simulink model "ros_test"  (R2025b)
settings: Solver=VariableStepAuto  StartTime=0.0  StopTime=inf  RelTol=1e-3
libraries: ros2lib x3
settings Model: Creator=vulcangrip  LastModifiedBy=cyclone

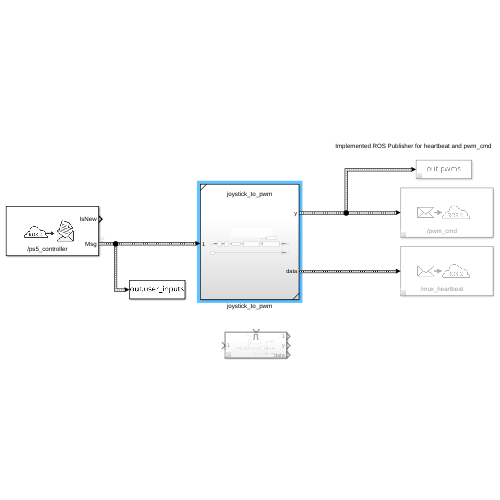
[thumbnail: Simulink's stored preview of the top-level diagram]
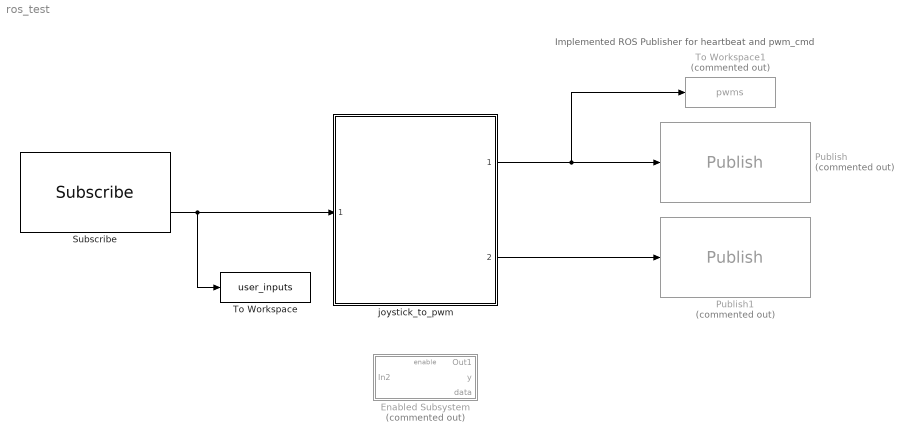
== system ros_test ==
  note: Implemented ROS Publisher for heartbeat and pwm_cmd
  Enabled Subsystem : Subsystem  Commented=on  TreatAsAtomicUnit=on
  Publish : ros2lib/Publish  Commented=on  topicSource=Specify your own  topic=/pwm_cmd  messageType=custom_interfaces/Pwms  QOSHistory=Keep last  QOSDepth=10  QOSReliability=Reliable  QOSDurability=Volatile  QOSDeadline=Inf  QOSLifespan=Inf  QOSLiveliness=Automatic  QOSLeaseDuration=Inf  QOSAvoidROSNamespaceConventions=off
  Publish1 : ros2lib/Publish  Commented=on  topicSource=Specify your own  topic=/mux_heartbeat  messageType=std_msgs/Bool  QOSHistory=Keep last  QOSDepth=10  QOSReliability=Reliable  QOSDurability=Volatile  QOSDeadline=Inf  QOSLifespan=Inf  QOSLiveliness=Automatic  QOSLeaseDuration=Inf  QOSAvoidROSNamespaceConventions=off
  Subscribe : ros2lib/Subscribe  topicSource=Specify your own  topic=/ps5_controller  messageType=remote_control_interface/Gamepad  sampleTime=1  QOSHistory=Keep last  QOSDepth=10  QOSReliability=Reliable  QOSDurability=Volatile  QOSDeadline=Inf  QOSLifespan=Inf  QOSLiveliness=Automatic  QOSLeaseDuration=Inf  QOSAvoidROSNamespaceConventions=off
  To Workspace : ToWorkspace  VariableName=user_inputs  SaveFormat=Timeseries  SampleTime=-1
  To Workspace1 : ToWorkspace  Commented=on  VariableName=pwms  SaveFormat=Timeseries  SampleTime=-1
  joystick_to_pwm : Subsystem  ReferencedSubsystem=joystick_to_pwm
  wires:
  Subscribe/2 -> To Workspace/1, joystick_to_pwm/1
  joystick_to_pwm/1 -> Publish/1, To Workspace1/1
  joystick_to_pwm/2 -> Publish1/1

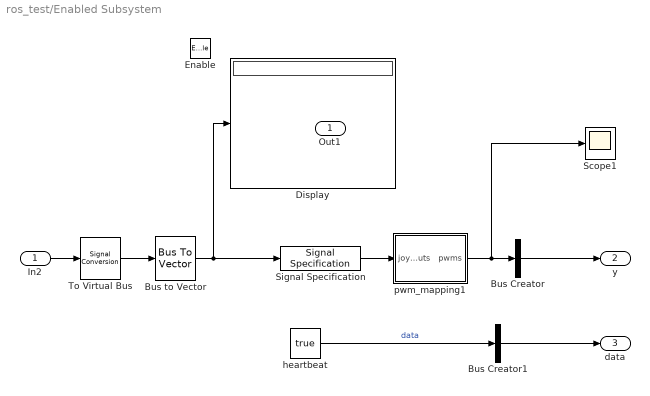
== system ros_test/Enabled Subsystem ==
  In2 : Inport
  Enable : EnablePort
  Bus Creator : BusCreator  Inputs=1  OutDataTypeStr=Bus: SL_Bus_custom_interfaces_Pwms  NonVirtualBus=on
  Bus Creator1 : BusCreator  Inputs=1  OutDataTypeStr=Bus: SL_Bus_std_msgs_Bool  NonVirtualBus=on
  Bus to Vector : BusToVector
  Display : Display
  Scope1 : Scope
      settings: ActiveDisplayYMinimum=-823919.38808281254  ActiveDisplayYMaximum=486800.61191718746
  Signal Specification : SignalSpecification  Dimensions=[6,1]
  To Virtual Bus : SignalConversion  ConversionOutput=Virtual bus  OverrideOpt=off
  heartbeat : Constant  Value=true
  pwm_mapping1 : MATLAB Function  TreatAsAtomicUnit=on
  Out1 : Outport
  y : Outport  Port=2
  data : Outport  Port=3
  wires:
  heartbeat/1 -> Bus Creator1/1  "data"
  In2/1 -> To Virtual Bus/1
  Signal Specification/1 -> pwm_mapping1/1(joystick_inputs)
  Bus to Vector/1 -> Signal Specification/1, Display/1
  Bus Creator/1 -> y/1
  Bus Creator1/1 -> data/1
  pwm_mapping1/1(pwms) -> Scope1/1, Bus Creator/1
  To Virtual Bus/1 -> Bus to Vector/1

== matlab function ros_test/Enabled Subsystem/pwm_mapping1 ==
  data: joystick_inputs input; pwms output
function pwms = fcn(joystick_inputs)

x = joystick_inputs(1);
y = joystick_inputs(2);
pitch = joystick_inputs(3);
yaw = joystick_inputs(4);
sink = joystick_inputs(5);
rise = joystick_inputs(6);
%Need to input the other 4, rise and sink as well as pitch and yaw

pwms = int32(zeros(8,1));
pwms(1) = int32(1500 + 60*x); %Thruster 0
pwms(2) = int32(1500 + 60*rise); %Thruster 4
pwms(3) = int32(1500 + 60*rise); %Thruster 5
pwms(4) = int32(1500 + 60*x); %Thruster 1
pwms(5) = int32(1500 + 60*rise); %Thruster ?
pwms(6) = int32(1500 + 60*x); %Thruster 3
pwms(7) = int32(1500 + 60*rise); %Thruster 7
pwms(8) = int32(1500 + 60*x); %Thruster 2


%Create the mapping here for PWM values.
%Recall that PWM 1-8 correspond to thruster postions which follow,

%pwm of each thruster on the robot
%In left to right:
%f = front / r = rear
%l = left  / r = right
%t = top   / b = bottom
%PWM(1)=pwm_flt
%PWM(2)=pwm_frt
%PWM(3)=pwm_rlt
%PWM(4)=pwm_rrt
%PWM(5)=pwm_flb
%PWM(6)=pwm_frb
%PWM(7)=pwm_rlb
%PWM(8)=pwm_rrb
